simulink model "KrisztaSimulink"  (R2023b)
settings: Solver=VariableStepAuto  StartTime=0.0  StopTime=10^6  RelTol=1e-3
settings Model: Creator=kBen  LastModifiedBy=kBen
settings SolverCC: AlgebraicLoopSolver=TrustRegion

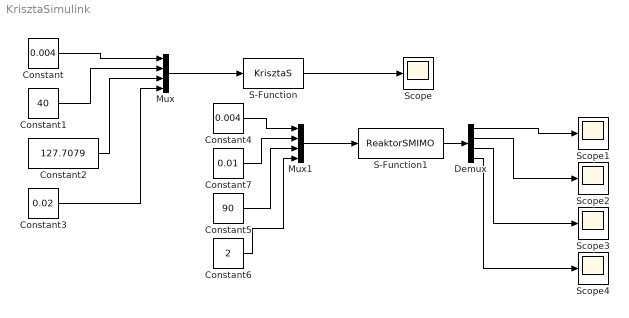
== system KrisztaSimulink ==
  Constant : Constant  Value=0.004
  Constant1 : Constant  Value=40
  Constant2 : Constant  Value=127.7079
  Constant3 : Constant  Value=0.02
  Constant4 : Constant  Value=0.004
  Constant5 : Constant  Value=90
  Constant6 : Constant  Value=2
  Constant7 : Constant  Value=0.01
  Demux : Demux
  Mux : Mux
  Mux1 : Mux
  S-Function : S-Function  FunctionName=KrisztaS  SFunctionDeploymentMode=off  EnableBusSupport=off
  S-Function1 : S-Function  FunctionName=ReaktorSMIMO  SFunctionDeploymentMode=off  EnableBusSupport=off
  Scope{,1..4} (5 alike) : Scope
  wires:
  Mux/1 -> S-Function/1
  S-Function/1 -> Scope/1
  Constant/1 -> Mux/1
  Constant1/1 -> Mux/2
  Constant2/1 -> Mux/3
  Constant3/1 -> Mux/4
  Mux1/1 -> S-Function1/1
  Constant4/1 -> Mux1/1
  Constant7/1 -> Mux1/2
  Constant5/1 -> Mux1/3
  Constant6/1 -> Mux1/4
  S-Function1/1 -> Demux/1
  Demux/1 -> Scope1/1
  Demux/2 -> Scope2/1
  Demux/3 -> Scope3/1
  Demux/4 -> Scope4/1
